simulink model "PR_sim_bahn_dreieck_freiflug"  (R2023b)
settings: Solver=FixedStepAuto  StartTime=0.0  StopTime=Te  FixedStep=Ts  RelTol=1e-3  EnableMultiTasking=on
settings Model: Creator=Hoebarth  LastModifiedBy=Flo
settings SolverCC: AlgebraicLoopSolver=TrustRegion
settings DataIOCC: LimitDataPoints=on  SaveFormat=Array  SignalLoggingSaveFormat=ModelDataLogs  ReturnWorkspaceOutputs=off
settings OptimizationCC: LifeSpan=inf
settings DebuggingCC: SaveWithParameterizedLinksMsg=none  UnderspecifiedInitializationDetection=Classic  MergeDetectMultiDrivingBlocksExec=none  SignalResolutionControl=TryResolveAllWithWarning  MultiTaskDSMMsg=warning  MultiTaskCondExecSysMsg=none  UnconnectedInputMsg=warning  UnconnectedOutputMsg=warning  UnconnectedLineMsg=warning  SFUnexpectedBacktrackingDiag=warning  SFNoUnconditionalDefaultTransitionDiag=warning  SFExecutionAtInitializationDiag=none  ArithmeticOperatorsInVariantConditions=warning
settings HardwareCC: ProdBitPerPointer=32  ProdBitPerSizeT=32  ProdBitPerPtrDiffT=32  ProdLargestAtomicFloat=None  ProdIntDivRoundTo=Undefined  ProdEndianess=Unspecified  ProdWordSize=32  ProdHWDeviceType=32-bit Generic  TargetUnknown=on
settings ModelReferenceCC: EnableRefExpFcnMdlSchedulingChecks=on  PropagateSignalLabelsOutOfModel=off
settings SFSimCC: SimUseLocalCustomCode=off  SimParseCustomCode=off  CustomCodeUndefinedFunction=UseInterfaceOnly
settings RTWCC: RTWUseLocalCustomCode=off
settings CodeAppCC: StateflowObjectComments=on
settings GRTTargetCC: TargetFcnLib=ansi_tfl_tmw.mat  TargetLangStandard=C89/C90 (ANSI)  CombineOutputUpdateFcns=off  GRTInterface=on
settings ConfigComp: CovMetricSettings=dw  CovSaveCumulativeToWorkspaceVar=on  CovSaveSingleToWorkspaceVar=on  CovExternalEMLEnable=off

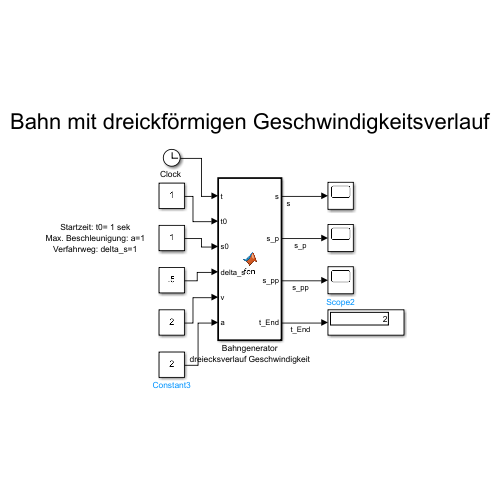
[thumbnail: Simulink's stored preview of the top-level diagram]
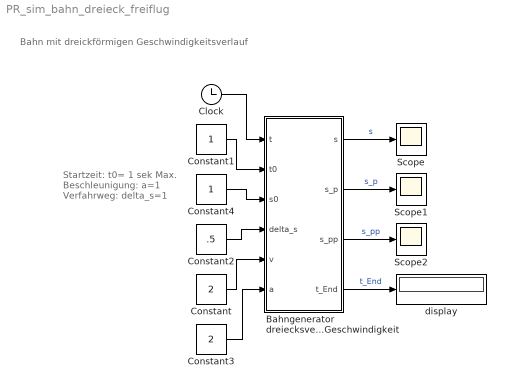
== system PR_sim_bahn_dreieck_freiflug ==
  note: Bahn mit dreickförmigen Geschwindigkeitsverlauf
  note: Startzeit: t0= 1 sek
      | Max. Beschleunigung: a=1
      | Verfahrweg: delta_s=1
  Bahngenerator dreiecksverlauf Geschwindigkeit : MATLAB Function  TreatAsAtomicUnit=on
  "Clock " : Clock
  Constant : Constant  Value=2
  Constant1 : Constant
  Constant2 : Constant  Value=.5
  Constant3 : Constant  Value=2
  Constant4 : Constant
  Scope : Scope
  Scope1 : Scope
  Scope2 : Scope
  display : Display
  wires:
  "Clock "/1 -> Bahngenerator dreiecksverlauf Geschwindigkeit/1(t)
  Constant1/1 -> Bahngenerator dreiecksverlauf Geschwindigkeit/2(t0)
  Constant4/1 -> Bahngenerator dreiecksverlauf Geschwindigkeit/3(s0)
  Bahngenerator dreiecksverlauf Geschwindigkeit/4(t_End) -> display/1  "t_End"
  Bahngenerator dreiecksverlauf Geschwindigkeit/2(s_p) -> Scope1/1  "s_p"
  Bahngenerator dreiecksverlauf Geschwindigkeit/1(s) -> Scope/1  "s"
  Bahngenerator dreiecksverlauf Geschwindigkeit/3(s_pp) -> Scope2/1  "s_pp"
  Constant2/1 -> Bahngenerator dreiecksverlauf Geschwindigkeit/4(delta_s)
  Constant3/1 -> Bahngenerator dreiecksverlauf Geschwindigkeit/6(a)
  Constant/1 -> Bahngenerator dreiecksverlauf Geschwindigkeit/5(v)

== matlab function PR_sim_bahn_dreieck_freiflug/Bahngenerator dreiecksverlauf Geschwindigkeit ==
  data: t input; s output; t0 input; s0 input; delta_s input; v input; a input; s_p output; s_pp output; t_End output
function [s, s_p, s_pp, t_End] = fcn(t, t0, s0, delta_s, v, a)
%#codegen

% Mein erster Bahngenerator:
% in embeded Matlab functions kann mit gewoehnlichem m-Code (Matlab Code)
% gearbeitet werden.

% todo: Implementierung Bahngenerator

tb = v / a;
tfrei = (-v*tb + abs(delta_s))/v;
Ta = 2 * sqrt(abs(delta_s)/a);
if tfrei > 0
    if t < t0
        s = 0;
        s_p = 0;
        s_pp = 0;
    elseif t < t0 + tb
        s = a/2 * (-t0 + t)^2;
        s_p = a * (t - t0);
        s_pp = a;
    elseif t < t0 + tb + tfrei
        s = a/2 * tb * (2*t - tb - 2*t0);
        s_p = a * (tb);
        s_pp = 0;
    elseif t < t0 + 2*tb + tfrei
        s = a*(-tb^2 + (2*t - 2*t0 -tfrei)*tb - (-t0 - tfrei +t)^2 /2);
        s_p = a * (t0 + 2*tb +tfrei - t);
        s_pp = -a;
    else
        s = a*tb*(tb +tfrei);
        s_p = 0;
        s_pp = 0;
    end
    t_End = t0 + 2*tb + tfrei;
else
    if t < t0
        s = 0;
        s_p = 0;
        s_pp = 0;
    elseif t < t0 + Ta/2
        s = a/2 * (-t0 + t)^2;
        s_p = a * (t - t0);
        s_pp = a;
    elseif t < t0 + Ta
        s = a/2 * (-Ta^2 / 2 + 2*(t - t0)*Ta - (t - t0)^2);
        s_p = a * (t0 + Ta - t);
        s_pp = -a;
    else
        s = a*Ta^2/4;
        s_p = 0;
        s_pp = 0;
    end
   
    t_End = t0 + Ta;
end
s = s * sign(delta_s) + s0;
s_p = s_p * sign(delta_s);
s_pp = s_pp * sign(delta_s);
